simulink model "rtwdemo_memsec"  (Simulink 7.6)
settings: Solver=FixedStepDiscrete  StartTime=0.0  StopTime=12.0  FixedStep=1  RelTol=1e-3
libraries: rtwdemowidgets x1
Description:
  | Memory Sections for Generated Functions and Data
settings Model: Creator=The MathWorks Inc.  ExtModeAutoUpdateStatusClock=off
settings MATStruct: SampleTime=1  Offset=0  Priority=[20.0]
settings DataIOCC: SaveOutput=off  SaveTime=off
settings OptimizationCC: InlineParams=on  InlineInvariantSignals=on  PassReuseOutputArgsAs=Individual arguments  StateBitsets=on  DataBitsets=on  UseTempVars=on  ZeroExternalMemoryAtStartup=off  ZeroInternalMemoryAtStartup=off  NoFixptDivByZeroProtection=on  EfficientFloat2IntCast=on  EfficientMapNaN2IntZero=off  OptimizeModelRefInitCode=on  LifeSpan=1
settings DebuggingCC: SolverPrmCheckMsg=none  StrictBusMsg=ErrorOnBusTreatedAsVector
settings HardwareCC: ProdIntDivRoundTo=Zero  ProdEndianess=LittleEndian  ProdHWDeviceType=Generic->32-bit Embedded Processor  TargetHWDeviceType=Generic->32-bit Embedded Processor
settings RTWCC: SystemTargetFile=ert.tlc  GenCodeOnly=on  TemplateMakefile=ert_default_tmf  Description=Real-Time Workshop Embedded Coder (no auto configuration)  GenerateReport=on  RTWVerbose=off  ProcessScript=ert_make_rtw_hook  IncludeHyperlinkInReport=on  LaunchReport=on
settings CodeAppCC: ForceParamTrailComments=on  IgnoreCustomStorageClasses=off  IgnoreTestpoints=on  SimulinkDataObjDesc=on  CustomSymbolStrGlobalVar=rt$N$M  CustomSymbolStrType=$N$M  CustomSymbolStrFcn=$N$M$F  CustomSymbolStrMacro=$N$M  InsertBlockDesc=on
settings ERTTargetCC: TargetFcnLib=ansi_tfl_tmw.mat  MultiwordLength=2048  GenerateSampleERTMain=on  IncludeMdlTerminateFcn=off  SupportNonFinite=off  SupportComplex=off  InlinedParameterPlacement=NonHierarchical  ERTCustomFileTemplate=example_file_process.tlc  ConvertIfToSwitch=off  MemSecPackage=ECoderDemos  MemSecDataConstants=MediumMemory  MemSecDataIO=MediumMemory  MemSecDataInternal=MediumMemory  MemSecDataParameters=MediumMemory  MemSecFuncInitTerm=MediumMemory  MemSecFuncExecute=MediumMemory

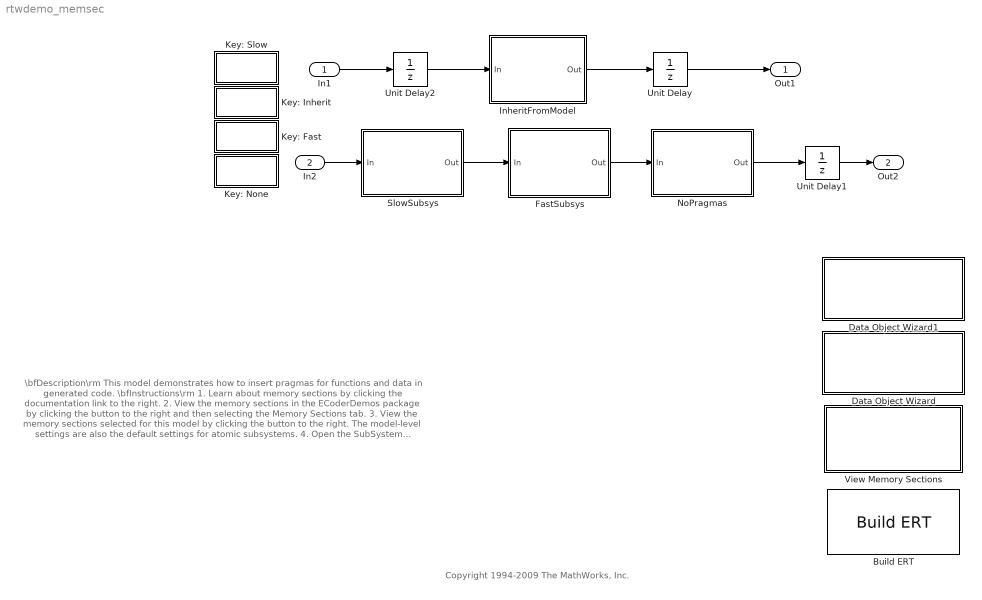
== system rtwdemo_memsec ==
  note: \bfDescription\rm
      | This model demonstrates how to insert pragmas for functions and data in generated code.
      |
      | \bfInstructions\rm
      | 1. Learn about memory sections by clicking the documentation link to the right.
      |
      | 2. View the memory sections in the ECoderDemos package by clicking the button
      |     to the right and then selecting the Memory Sections tab.
      |
      | 3. View the memory sections selected for this model by clicking the button to the right.
      |     The model-level settings are also the default settings for atomic subsystems.
      |
      | 4. Open the SubSystem Parameters dialog for the subsystems to see the
      |     memory section settings for each of the atomic subsystems in this model.
      |
      | 5. Generate code by clicking the button to the right.  An HTML report is displayed
      |     automatically.  Inspect the data and function definitions in the .c files and observe
      |     how the generated pragmas correspond to the selected memory sections.
  note: Copyright 1994-2009 The MathWorks, Inc.
  In1 : Inport  OutDataTypeStr=double  PortDimensions=1  SampleTime=1
  In2 : Inport  Port=2  OutDataTypeStr=double  PortDimensions=1  SampleTime=1
  " View Memory Sections" : Subsystem
      settings: OpenFcn=|
      | if ecoderinstalled
      | 
      | dlg = slCfgPrmDlg(bdroot,'Open');
      | dlg = slCfgPrmDlg(bdroot,'TurnToPage','Memory Sections'); clear dlg;
      | 
      | else
      | 
      | errordlg(sprintf('This demo requires Real-Time Workshop Embedded Coder.'))
      | 
      | end
      mask Display: disp('Memory Sections\nFor This Model\n(double-click)')
  Build ERT : rtwdemowidgets/Build ERT  SystemSampleTime=-1  attrib_overrides={'MemSecPackage'; 'MemSecDataConstants'; 'MemSecDataIO'; 'MemSecDataInternal'; 'MemSecDataParameters'; 'MemSecFuncInitTerm'; 'MemSecFuncExecute'; 'ERTFilePackagingFormat'}
  Data Object Wizard : Subsystem  Description=cscdesigner
      settings: OpenFcn=|
      | if ecoderinstalled
      | 
      | cscdesigner ECoderDemos
      | 
      | else
      | 
      | errordlg(sprintf('This demo requires Real-Time Workshop Embedded Coder.'))
      | 
      | end
      mask Type: Custom storage class designer
      mask Description: Custom storage class designer for defining custom storage classes and memory sections inside a package.
      mask Help: helpview([docroot,'/toolbox/ecoder/helptargets.map'],'data_obj_wiz');
      mask Display: disp('Memory Section\nDefinitions\n(double-click)');
  Data Object Wizard1 : Subsystem  Description=User documentation
      settings: OpenFcn=|
      | if ecoderinstalled
      | 
      | helpview([docroot '/toolbox/ecoder/helptargets.map'], 'memsects')
      | 
      | else
      | 
      | errordlg(sprintf('This demo requires Real-Time Workshop Embedded Coder.'))
      | 
      | end
      mask Type: Memory section documentation
      mask Description: Memory section documentation
      mask Display: disp('View User\nDocumentation\n(double-click)')
  FastSubsys : Subsystem  TreatAsAtomicUnit=on
      settings: RTWSystemCode=Function  RTWFileNameOpts=Use subsystem name  FunctionWithSeparateData=on  RTWMemSecFuncInitTerm=FastMemory  RTWMemSecFuncExecute=FastMemory  RTWMemSecDataConstants=FastMemory  RTWMemSecDataInternal=FastMemory  RTWMemSecDataParameters=FastMemory
  InheritFromModel : Subsystem  TreatAsAtomicUnit=on
      settings: RTWSystemCode=Function  RTWFileNameOpts=Use subsystem name  FunctionWithSeparateData=on
  Key: Fast : Subsystem  TreatAsAtomicUnit=on
      settings: RTWSystemCode=Function  FunctionWithSeparateData=on
      mask Display: disp('Fast')
  Key: Inherit : Subsystem  TreatAsAtomicUnit=on
      settings: RTWSystemCode=Function  FunctionWithSeparateData=on
      mask Display: disp('Inherit')
  Key: None : Subsystem  TreatAsAtomicUnit=on
      settings: RTWSystemCode=Function  FunctionWithSeparateData=on
      mask Display: disp('None')
  Key: Slow : Subsystem  TreatAsAtomicUnit=on
      settings: RTWSystemCode=Function  FunctionWithSeparateData=on
      mask Display: disp('Slow')
  NoPragmas : Subsystem  TreatAsAtomicUnit=on
      settings: RTWSystemCode=Function  RTWFileNameOpts=Use subsystem name  FunctionWithSeparateData=on  RTWMemSecFuncInitTerm=Default  RTWMemSecFuncExecute=Default  RTWMemSecDataConstants=Default  RTWMemSecDataInternal=Default  RTWMemSecDataParameters=Default
  SlowSubsys : Subsystem  TreatAsAtomicUnit=on
      settings: RTWSystemCode=Function  RTWFileNameOpts=Use subsystem name  FunctionWithSeparateData=on  RTWMemSecFuncInitTerm=SlowMemory  RTWMemSecFuncExecute=SlowMemory  RTWMemSecDataConstants=SlowMemory  RTWMemSecDataInternal=SlowMemory  RTWMemSecDataParameters=SlowMemory
  Unit Delay : UnitDelay
  Unit Delay1 : UnitDelay
  Unit Delay2 : UnitDelay
  Out1 : Outport
  Out2 : Outport  Port=2
  wires:
  In2/1 -> SlowSubsys/1(In)
  FastSubsys/1(Out) -> NoPragmas/1(In)
  In1/1 -> Unit Delay2/1
  InheritFromModel/1(Out) -> Unit Delay/1
  SlowSubsys/1(Out) -> FastSubsys/1(In)
  NoPragmas/1(Out) -> Unit Delay1/1
  Unit Delay/1 -> Out1/1
  Unit Delay1/1 -> Out2/1
  Unit Delay2/1 -> InheritFromModel/1(In)

== system rtwdemo_memsec/ View Memory Sections ==

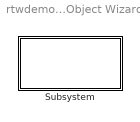
== system rtwdemo_memsec/Data Object Wizard ==
  Subsystem : Subsystem

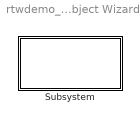
== system rtwdemo_memsec/Data Object Wizard1 ==
  Subsystem : Subsystem

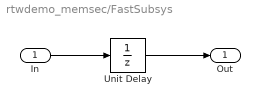
== system rtwdemo_memsec/FastSubsys ==
  In : Inport
  "Unit Delay " : UnitDelay
  Out : Outport
  wires:
  In/1 -> "Unit Delay "/1
  "Unit Delay "/1 -> Out/1

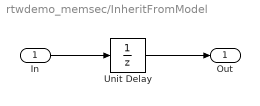
== system rtwdemo_memsec/InheritFromModel ==
  In : Inport
  Unit Delay : UnitDelay
  Out : Outport
  wires:
  Unit Delay/1 -> Out/1
  In/1 -> Unit Delay/1

== system rtwdemo_memsec/Key: Fast ==
  note: The "FastMemory" memory section is defined to generate the following
      | comment and pragma before the relevant functions and data:
  note: /* This memory is fast but expensive */
      | #pragma FAST_MEM(%<identifier>)

== system rtwdemo_memsec/Key: Inherit ==
  note: The model is configured to generate its functions and data into "MediumMemory".
      | As a result, the following comment and pragma are generated before the model's
      | functions and data.  Unless otherwise specified, subsystems use the same
      | memory sections as the model ('Inherit from model').
  note: /* This memory is of moderate speed and cost */
      | #pragma MEDIUM_MEM(%<identifier>)

== system rtwdemo_memsec/Key: None ==
  note: The "Default" memory section does not generate any comments or
      | pragmas around the corresponding functions and data.

== system rtwdemo_memsec/Key: Slow ==
  note: The "SlowMemory" memory section is defined to generate the following
      | comment and pragma before the relevant functions and data:
  note: /* This memory is cheap but slow */
      | #pragma SLOW_MEM(%<identifier>)

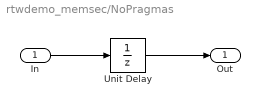
== system rtwdemo_memsec/NoPragmas ==
  In : Inport
  Unit Delay : UnitDelay
  Out : Outport
  wires:
  In/1 -> Unit Delay/1
  Unit Delay/1 -> Out/1

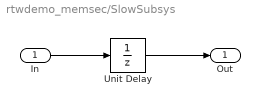
== system rtwdemo_memsec/SlowSubsys ==
  In : Inport
  Unit Delay : UnitDelay
  Out : Outport
  wires:
  In/1 -> Unit Delay/1
  Unit Delay/1 -> Out/1

== system rtwdemo_memsec/Data Object Wizard/Subsystem ==

== system rtwdemo_memsec/Data Object Wizard1/Subsystem ==
